simulink model "RBD_sim_model"  (R2023b)
settings: Solver=ode4  StartTime=t0  StopTime=tf  FixedStep=dt  RelTol=1e-3
values from neighbouring files (symbols this model uses):
  Forces = [2; 8; 3]    [get_forces_and_moments.m]
  Moments = [14; 20; 7]    [get_forces_and_moments.m]
undefined symbols (not defined in the file or in its folder): p0, phi0, psi0, q0, r0, theta0, u0, v0, w0, x0, y_0, z0
libraries: shared6dof x1, dspsigops x1
settings Model: Creator=Ahmed Raamadan  LastModifiedBy=Ahmed Raamadan

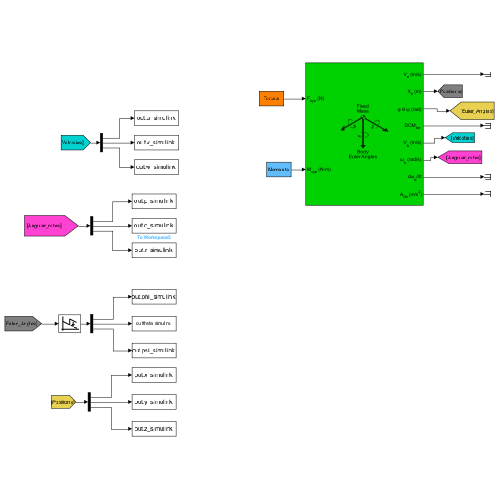
[thumbnail: Simulink's stored preview of the top-level diagram]
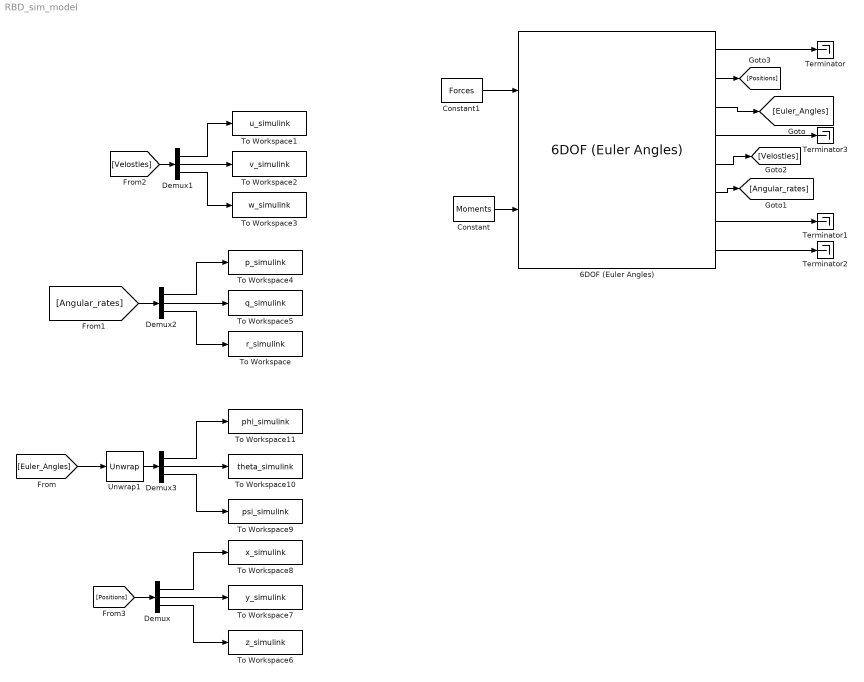
== system RBD_sim_model ==
  6DOF (Euler Angles) : shared6dof/6DOF (Euler Angles)  units=Metric (MKS)  mtype=Fixed  rep=Euler Angles  xme_0=[x0 y_0 z0]  Vm_0=[u0 v0 w0]  eul_0=[phi0 theta0 psi0]  pm_0=[p0 q0 r0]  mass_0=m  mass_e=0.5  mass_f=2.0  inertia=I_mat  inertia_e=eye(3)  inertia_f=2*eye(3)  k_quat=1.0  vre_flag=on  abi_flag=off  aMode=0  xme_statename=''  Vm_statename=''  eul_statename=''  quat_statename=''  pm_statename=''  mass_statename=''
  Constant : Constant  Value=Moments
  Constant1 : Constant  Value=Forces
  Demux{,1..3} (4 alike) : Demux  Outputs=3
  Terminator{,1..3} (4 alike) : Terminator
  To Workspace : ToWorkspace  VariableName=r_simulink  SaveFormat=Timeseries  SampleTime=-1
  To Workspace1 : ToWorkspace  VariableName=u_simulink  SaveFormat=Timeseries  SampleTime=-1
  To Workspace10 : ToWorkspace  VariableName=theta_simulink  SaveFormat=Timeseries  SampleTime=-1
  To Workspace11 : ToWorkspace  VariableName=phi_simulink  SaveFormat=Timeseries  SampleTime=-1
  To Workspace2 : ToWorkspace  VariableName=v_simulink  SaveFormat=Timeseries  SampleTime=-1
  To Workspace3 : ToWorkspace  VariableName=w_simulink  SaveFormat=Timeseries  SampleTime=-1
  To Workspace4 : ToWorkspace  VariableName=p_simulink  SaveFormat=Timeseries  SampleTime=-1
  To Workspace5 : ToWorkspace  VariableName=q_simulink  SaveFormat=Timeseries  SampleTime=-1
  To Workspace6 : ToWorkspace  VariableName=z_simulink  SaveFormat=Timeseries  SampleTime=-1
  To Workspace7 : ToWorkspace  VariableName=y_simulink  SaveFormat=Timeseries  SampleTime=-1
  To Workspace8 : ToWorkspace  VariableName=x_simulink  SaveFormat=Timeseries  SampleTime=-1
  To Workspace9 : ToWorkspace  VariableName=psi_simulink  SaveFormat=Timeseries  SampleTime=-1
  Unwrap1 : dspsigops/Unwrap  tol=pi  running=off
  wires:
  6DOF (Euler Angles)/1 -> Terminator/1
  6DOF (Euler Angles)/7 -> Terminator1/1
  6DOF (Euler Angles)/8 -> Terminator2/1
  Demux/1 -> To Workspace8/1
  Demux/2 -> To Workspace7/1
  Demux/3 -> To Workspace6/1
  Demux1/1 -> To Workspace1/1
  Demux1/3 -> To Workspace3/1
  Demux1/2 -> To Workspace2/1
  Demux2/1 -> To Workspace4/1
  Demux2/2 -> To Workspace5/1
  Demux2/3 -> To Workspace/1
  Demux3/3 -> To Workspace9/1
  Demux3/2 -> To Workspace10/1
  Demux3/1 -> To Workspace11/1
  Constant/1 -> 6DOF (Euler Angles)/2
  Constant1/1 -> 6DOF (Euler Angles)/1
  6DOF (Euler Angles)/4 -> Terminator3/1
  6DOF (Euler Angles)/6 -> [Angular_rates]
  6DOF (Euler Angles)/3 -> [Euler_Angles]
  [Euler_Angles] -> Unwrap1/1
  Unwrap1/1 -> Demux3/1
  [Angular_rates] -> Demux2/1
  6DOF (Euler Angles)/5 -> [Velosties]
  [Velosties] -> Demux1/1
  6DOF (Euler Angles)/2 -> [Positions]
  [Positions] -> Demux/1
